simulink model "manual_PID"  (R2023b)
settings: Solver=VariableStepAuto  StartTime=0.0  StopTime=10.0  RelTol=1e-3
undefined symbols (not defined in the file): c, g, m
settings Model: Creator=Jack  LastModifiedBy=Jack

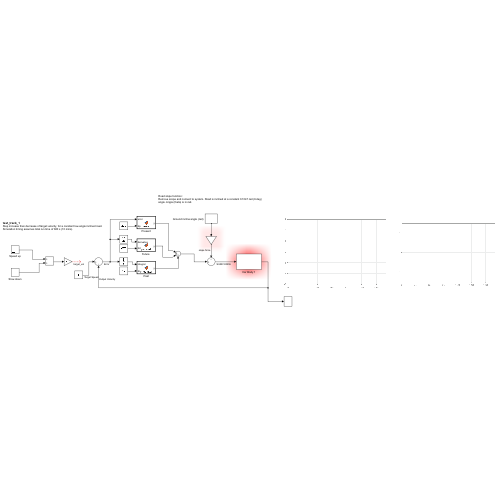
[thumbnail: Simulink's stored preview of the top-level diagram]
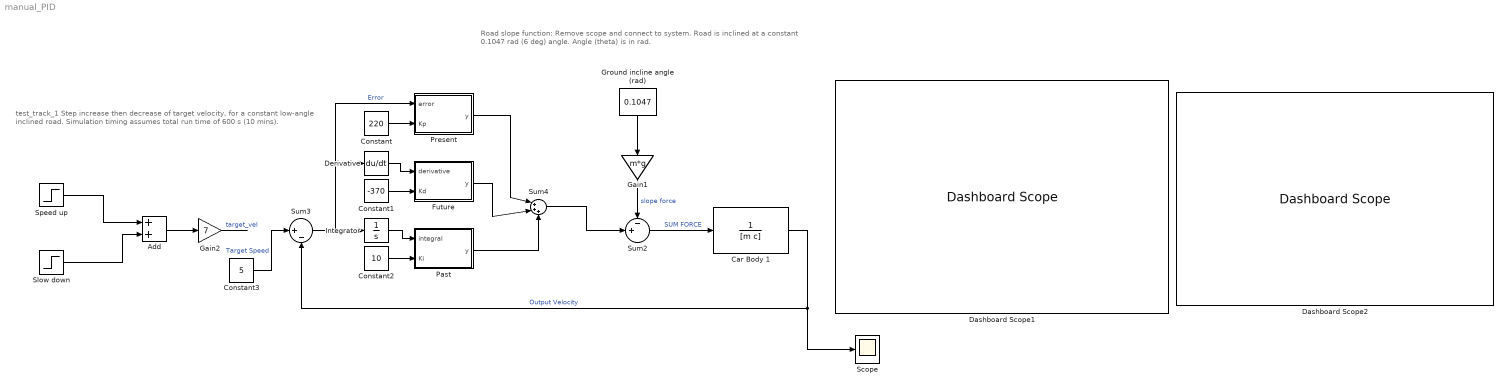
== system manual_PID ==
  note: Road slope function:
      | Remove scope and connect to system. Road is inclined at a constant 0.1047 rad (6 deg) angle. Angle (theta) is in rad.
  note: test_track_1
      | Step increase then decrease of target velocity, for a constant low-angle inclined road.
      | Simulation timing assumes total run time of 600 s (10 mins).
  Add : Sum
  Car Body 1 : TransferFcn  Denominator=[m c]
  Constant : Constant  Value=220
  Constant1 : Constant  Value=-370
  Constant2 : Constant  Value=10
  Constant3 : Constant  Value=5
  Dashboard Scope1 : DashboardScope  TimeSpan=200  NormalizeYAxis=on
  Dashboard Scope2 : DashboardScope  TimeSpan=200  NormalizeYAxis=on
  Derivative : Derivative
  "Future " : MATLAB Function  TreatAsAtomicUnit=on
  Gain1 : Gain  Gain=m*g
  Gain2 : Gain  Gain=7
  Ground incline angle (rad) : Constant  Value=0.1047
  Integrator : Integrator
  Past : MATLAB Function  TreatAsAtomicUnit=on
  Present : MATLAB Function  TreatAsAtomicUnit=on
  Scope : Scope
  Slow down : Step  Time=300  Before=3  After=2  SampleTime=0
  Speed up : Step  Time=50  Before=1  After=3  SampleTime=0
  Sum2 : Sum  Inputs=-+|
  Sum3 : Sum  Inputs=|+-
  Sum4 : Sum  Inputs=|+++
  wires:
  Gain2/1 -> ?  "target_vel"
  Ground incline angle (rad)/1 -> Gain1/1
  Speed up/1 -> Add/1
  Constant3/1 -> Sum3/1  "Target Speed"
  Constant1/1 -> "Future "/2(Kd)
  Sum3/1 -> Present/1(error), Derivative/1, Integrator/1  "Error"
  Sum4/1 -> Sum2/2
  Derivative/1 -> "Future "/1(derivative)
  Integrator/1 -> Past/1(integral)
  Constant/1 -> Present/2(Kp)
  Car Body 1/1 -> Scope/1, Sum3/2  "Output Velocity"
  Present/1(y) -> Sum4/1
  Constant2/1 -> Past/2(Ki)
  Slow down/1 -> Add/2
  "Future "/1(y) -> Sum4/2
  Add/1 -> Gain2/1
  Past/1(y) -> Sum4/3
  Sum2/1 -> Car Body 1/1  "SUM FORCE"
  Gain1/1 -> Sum2/1  "slope force"

== matlab function manual_PID/Past ==
  data: integral input; y output; Ki input
function y = integrator(integral, Ki)
    y = Ki * integral;
end

== matlab function manual_PID/Present ==
  data: error input; y output; Kp input
function y = Past(error, Kp)
    y = Kp * error;
end

== matlab function manual_PID/Future  ==
  data: derivative input; y output; Kd input
function y = present(derivative, Kd)
    y = Kd * derivative;
end
